simulink model "doc_rstrig"  (R2014a)
settings: Solver=FixedStepDiscrete  StartTime=0.0  StopTime=3  RelTol=1e-3
undefined symbols (not defined in the file or in its folder): rsgenpoly
libraries: commblkcod2 x4, commrandsrc2 x1, dspsrcs4 x1
settings Model: Creator=The MathWorks Inc.
settings DataIOCC: SignalLoggingSaveFormat=ModelDataLogs
settings OptimizationCC: ExpressionDepthLimit=2147483647  InitFltsAndDblsToZero=on
settings DebuggingCC: SaveWithParameterizedLinksMsg=none  UnderspecifiedInitializationDetection=Classic  SignalResolutionControl=TryResolveAllWithWarning  MultiTaskDSMMsg=warning  MultiTaskCondExecSysMsg=none  FcnCallInpInsideContextMsg=UseLocalSettings  StateNameClashWarn=warning  StrictBusMsg=None
settings RTWCC: IncludeERTFirstTime=on
settings GRTTargetCC: TargetFcnLib=ansi_tfl_tmw.mat  CombineOutputUpdateFcns=off  GRTInterface=on

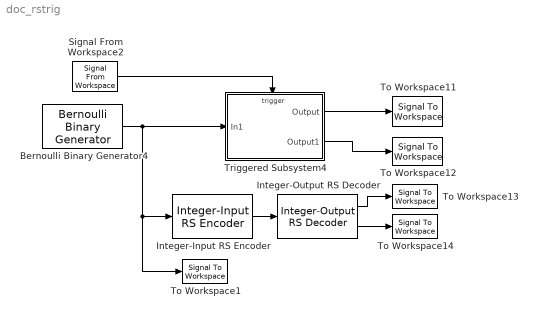
== system doc_rstrig ==
  Bernoulli Binary Generator4 : commrandsrc2/Bernoulli Binary Generator  P=0.5  seed=61  Ts=0.1  frameBased=on  sampPerFrame=3  orient=off  outDataType=double
  Integer-Input RS Encoder : commblkcod2/Integer-Input RS Encoder  n=7  k=3  specPrimPoly=off  prPoly=[1 0 1 1]  specGenPoly=off  genPoly=rsgenpoly(7,3)  specPuncture=off  punctVec=[ones(2,1); zeros(2,1)]
  Integer-Output RS Decoder : commblkcod2/Integer-Output RS Decoder  n=7  k=3  specPrimPoly=off  prPoly=[1 0 1 1]  specGenPoly=off  genPoly=rsgenpoly(7,3)  specPuncture=off  punctVec=[ones(2,1); zeros(2,1)]  specErasurePort=off  showNumErr=on
  Signal From Workspace2 : dspsrcs4/Signal From Workspace  X=[0 1]  Ts=0.3  nsamps=1  OutputAfterFinalValue=Cyclic repetition  ignoreOrWarnInputAndFrameLengths=off
  To Workspace1 : SignalToWorkspace  VariableName=input
  To Workspace11 : SignalToWorkspace  VariableName=trig_out
  To Workspace12 : SignalToWorkspace  VariableName=trig_out1
  To Workspace13 : SignalToWorkspace  VariableName=sim_out
  To Workspace14 : SignalToWorkspace  VariableName=sim_out1
  Triggered Subsystem4 : Subsystem  TreatAsAtomicUnit=on
  wires:
  Signal From Workspace2/1 -> Triggered Subsystem4/Trigger
  Bernoulli Binary Generator4/1 -> Triggered Subsystem4/1(In1), Integer-Input RS Encoder/1, To Workspace1/1
  Triggered Subsystem4/1(Output) -> To Workspace11/1
  Triggered Subsystem4/2(Output1) -> To Workspace12/1
  Integer-Input RS Encoder/1 -> Integer-Output RS Decoder/1
  Integer-Output RS Decoder/1 -> To Workspace13/1
  Integer-Output RS Decoder/2 -> To Workspace14/1

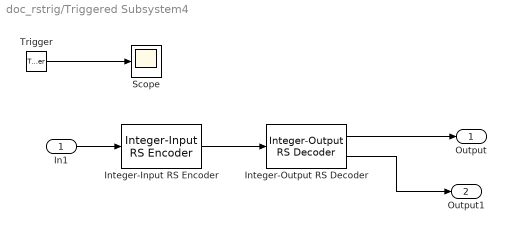
== system doc_rstrig/Triggered Subsystem4 ==
  In1 : Inport
  Trigger : TriggerPort  ShowOutputPort=on
  Integer-Input RS Encoder : commblkcod2/Integer-Input RS Encoder  n=7  k=3  specPrimPoly=off  prPoly=[1 0 1 1]  specGenPoly=off  genPoly=rsgenpoly(7,3)  specPuncture=off  punctVec=[ones(2,1); zeros(2,1)]
  Integer-Output RS Decoder : commblkcod2/Integer-Output RS Decoder  n=7  k=3  specPrimPoly=off  prPoly=[1 0 1 1]  specGenPoly=off  genPoly=rsgenpoly(7,3)  specPuncture=off  punctVec=[ones(2,1); zeros(2,1)]  specErasurePort=off  showNumErr=on
  Scope : Scope
  Output : Outport
  Output1 : Outport  Port=2
  wires:
  Integer-Input RS Encoder/1 -> Integer-Output RS Decoder/1
  Integer-Output RS Decoder/2 -> Output1/1
  In1/1 -> Integer-Input RS Encoder/1
  Integer-Output RS Decoder/1 -> Output/1
  Trigger/1 -> Scope/1
